simulink model "Thirtybussys_final"  (R2023b)
settings: Solver=VariableStepAuto  StartTime=0.0  StopTime=0.7  RelTol=1e-3
libraries: eePowerMeasurement x60, spsFourierLib x60, spsThreePhaseSeriesRLCBranchLib x41, spsThreePhaseVIMeasurementLib x30, spsThreePhaseSeriesRLCLoadLib x21, spsThreePhaseSourceLib x6, spsThreePhaseTransformerTwoWindingsLib x6, spsThreePhaseFaultLib x2, spspowerguiLib x1
(part 2 of 3)

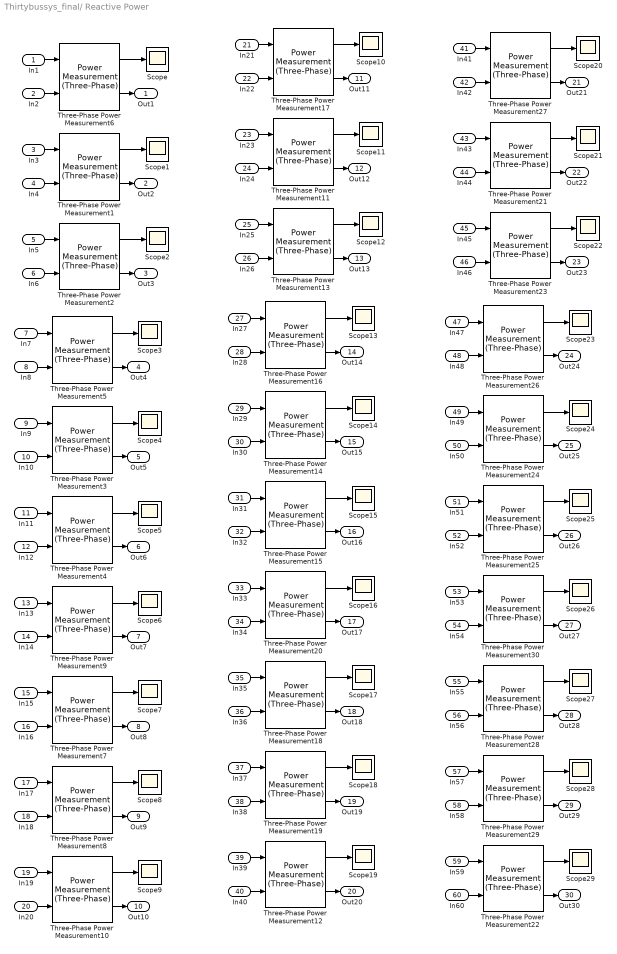
== system Thirtybussys_final/ Reactive Power ==
  In1 : Inport
  In2 : Inport  Port=2
  In3 : Inport  Port=3
  In4 : Inport  Port=4
  In5 : Inport  Port=5
  In6 : Inport  Port=6
  In7 : Inport  Port=7
  In8 : Inport  Port=8
  In9 : Inport  Port=9
  In10 : Inport  Port=10
  In11 : Inport  Port=11
  In12 : Inport  Port=12
  In13 : Inport  Port=13
  In14 : Inport  Port=14
  In15 : Inport  Port=15
  In16 : Inport  Port=16
  In17 : Inport  Port=17
  In18 : Inport  Port=18
  In19 : Inport  Port=19
  In20 : Inport  Port=20
  In21 : Inport  Port=21
  In22 : Inport  Port=22
  In23 : Inport  Port=23
  In24 : Inport  Port=24
  In25 : Inport  Port=25
  In26 : Inport  Port=26
  In27 : Inport  Port=27
  In28 : Inport  Port=28
  In29 : Inport  Port=29
  In30 : Inport  Port=30
  In31 : Inport  Port=31
  In32 : Inport  Port=32
  In33 : Inport  Port=33
  In34 : Inport  Port=34
  In35 : Inport  Port=35
  In36 : Inport  Port=36
  In37 : Inport  Port=37
  In38 : Inport  Port=38
  In39 : Inport  Port=39
  In40 : Inport  Port=40
  In41 : Inport  Port=41
  In42 : Inport  Port=42
  In43 : Inport  Port=43
  In44 : Inport  Port=44
  In45 : Inport  Port=45
  In46 : Inport  Port=46
  In47 : Inport  Port=47
  In48 : Inport  Port=48
  In49 : Inport  Port=49
  In50 : Inport  Port=50
  In51 : Inport  Port=51
  In52 : Inport  Port=52
  In53 : Inport  Port=53
  In54 : Inport  Port=54
  In55 : Inport  Port=55
  In56 : Inport  Port=56
  In57 : Inport  Port=57
  In58 : Inport  Port=58
  In59 : Inport  Port=59
  In60 : Inport  Port=60
  Scope{,1..29} (30 alike) : Scope
  Three-Phase Power Measurement{1..30} (30 alike) : eePowerMeasurement/Power Measurement (Three-Phase)  LabelModeActiveChoice=Continuous  F=60  K=0  Seq=Positive  Ts=0
  Out1 : Outport  VectorParamsAs1DForOutWhenUnconnected=off
  Out2 : Outport  Port=2  VectorParamsAs1DForOutWhenUnconnected=off
  Out3 : Outport  Port=3  VectorParamsAs1DForOutWhenUnconnected=off
  Out4 : Outport  Port=4  VectorParamsAs1DForOutWhenUnconnected=off
  Out5 : Outport  Port=5  VectorParamsAs1DForOutWhenUnconnected=off
  Out6 : Outport  Port=6  VectorParamsAs1DForOutWhenUnconnected=off
  Out7 : Outport  Port=7  VectorParamsAs1DForOutWhenUnconnected=off
  Out8 : Outport  Port=8  VectorParamsAs1DForOutWhenUnconnected=off
  Out9 : Outport  Port=9  VectorParamsAs1DForOutWhenUnconnected=off
  Out10 : Outport  Port=10  VectorParamsAs1DForOutWhenUnconnected=off
  Out11 : Outport  Port=11  VectorParamsAs1DForOutWhenUnconnected=off
  Out12 : Outport  Port=12  VectorParamsAs1DForOutWhenUnconnected=off
  Out13 : Outport  Port=13  VectorParamsAs1DForOutWhenUnconnected=off
  Out14 : Outport  Port=14  VectorParamsAs1DForOutWhenUnconnected=off
  Out15 : Outport  Port=15  VectorParamsAs1DForOutWhenUnconnected=off
  Out16 : Outport  Port=16  VectorParamsAs1DForOutWhenUnconnected=off
  Out17 : Outport  Port=17  VectorParamsAs1DForOutWhenUnconnected=off
  Out18 : Outport  Port=18  VectorParamsAs1DForOutWhenUnconnected=off
  Out19 : Outport  Port=19  VectorParamsAs1DForOutWhenUnconnected=off
  Out20 : Outport  Port=20  VectorParamsAs1DForOutWhenUnconnected=off
  Out21 : Outport  Port=21  VectorParamsAs1DForOutWhenUnconnected=off
  Out22 : Outport  Port=22  VectorParamsAs1DForOutWhenUnconnected=off
  Out23 : Outport  Port=23  VectorParamsAs1DForOutWhenUnconnected=off
  Out24 : Outport  Port=24  VectorParamsAs1DForOutWhenUnconnected=off
  Out25 : Outport  Port=25  VectorParamsAs1DForOutWhenUnconnected=off
  Out26 : Outport  Port=26  VectorParamsAs1DForOutWhenUnconnected=off
  Out27 : Outport  Port=27  VectorParamsAs1DForOutWhenUnconnected=off
  Out28 : Outport  Port=28  VectorParamsAs1DForOutWhenUnconnected=off
  Out29 : Outport  Port=29  VectorParamsAs1DForOutWhenUnconnected=off
  Out30 : Outport  Port=30  VectorParamsAs1DForOutWhenUnconnected=off
  wires:
  In2/1 -> Three-Phase Power Measurement6/2
  In1/1 -> Three-Phase Power Measurement6/1
  Three-Phase Power Measurement6/2 -> Out1/1
  Three-Phase Power Measurement6/1 -> Scope/1
  Three-Phase Power Measurement1/1 -> Scope1/1
  Three-Phase Power Measurement1/2 -> Out2/1
  In3/1 -> Three-Phase Power Measurement1/1
  In4/1 -> Three-Phase Power Measurement1/2
  In6/1 -> Three-Phase Power Measurement2/2
  In5/1 -> Three-Phase Power Measurement2/1
  Three-Phase Power Measurement2/2 -> Out3/1
  Three-Phase Power Measurement2/1 -> Scope2/1
  Three-Phase Power Measurement4/1 -> Scope5/1
  Three-Phase Power Measurement4/2 -> Out6/1
  In11/1 -> Three-Phase Power Measurement4/1
  In12/1 -> Three-Phase Power Measurement4/2
  In10/1 -> Three-Phase Power Measurement3/2
  In9/1 -> Three-Phase Power Measurement3/1
  Three-Phase Power Measurement3/2 -> Out5/1
  Three-Phase Power Measurement3/1 -> Scope4/1
  Three-Phase Power Measurement5/1 -> Scope3/1
  Three-Phase Power Measurement5/2 -> Out4/1
  In7/1 -> Three-Phase Power Measurement5/1
  In8/1 -> Three-Phase Power Measurement5/2
  In14/1 -> Three-Phase Power Measurement9/2
  In13/1 -> Three-Phase Power Measurement9/1
  Three-Phase Power Measurement9/2 -> Out7/1
  Three-Phase Power Measurement9/1 -> Scope6/1
  Three-Phase Power Measurement7/1 -> Scope7/1
  Three-Phase Power Measurement7/2 -> Out8/1
  In15/1 -> Three-Phase Power Measurement7/1
  In16/1 -> Three-Phase Power Measurement7/2
  In18/1 -> Three-Phase Power Measurement8/2
  In17/1 -> Three-Phase Power Measurement8/1
  Three-Phase Power Measurement8/2 -> Out9/1
  Three-Phase Power Measurement8/1 -> Scope8/1
  Three-Phase Power Measurement10/1 -> Scope9/1
  Three-Phase Power Measurement10/2 -> Out10/1
  In19/1 -> Three-Phase Power Measurement10/1
  In20/1 -> Three-Phase Power Measurement10/2
  In40/1 -> Three-Phase Power Measurement12/2
  In39/1 -> Three-Phase Power Measurement12/1
  Three-Phase Power Measurement12/2 -> Out20/1
  Three-Phase Power Measurement12/1 -> Scope19/1
  Three-Phase Power Measurement19/1 -> Scope18/1
  Three-Phase Power Measurement19/2 -> Out19/1
  In37/1 -> Three-Phase Power Measurement19/1
  In38/1 -> Three-Phase Power Measurement19/2
  In36/1 -> Three-Phase Power Measurement18/2
  In35/1 -> Three-Phase Power Measurement18/1
  Three-Phase Power Measurement18/2 -> Out18/1
  Three-Phase Power Measurement18/1 -> Scope17/1
  Three-Phase Power Measurement20/1 -> Scope16/1
  Three-Phase Power Measurement20/2 -> Out17/1
  In33/1 -> Three-Phase Power Measurement20/1
  In34/1 -> Three-Phase Power Measurement20/2
  In28/1 -> Three-Phase Power Measurement16/2
  In27/1 -> Three-Phase Power Measurement16/1
  Three-Phase Power Measurement16/2 -> Out14/1
  Three-Phase Power Measurement16/1 -> Scope13/1
  Three-Phase Power Measurement14/1 -> Scope14/1
  Three-Phase Power Measurement14/2 -> Out15/1
  In29/1 -> Three-Phase Power Measurement14/1
  In30/1 -> Three-Phase Power Measurement14/2
  In32/1 -> Three-Phase Power Measurement15/2
  In31/1 -> Three-Phase Power Measurement15/1
  Three-Phase Power Measurement15/2 -> Out16/1
  Three-Phase Power Measurement15/1 -> Scope15/1
  Three-Phase Power Measurement13/1 -> Scope12/1
  Three-Phase Power Measurement13/2 -> Out13/1
  In25/1 -> Three-Phase Power Measurement13/1
  In26/1 -> Three-Phase Power Measurement13/2
  In24/1 -> Three-Phase Power Measurement11/2
  In23/1 -> Three-Phase Power Measurement11/1
  Three-Phase Power Measurement11/2 -> Out12/1
  Three-Phase Power Measurement11/1 -> Scope11/1
  Three-Phase Power Measurement17/1 -> Scope10/1
  Three-Phase Power Measurement17/2 -> Out11/1
  In21/1 -> Three-Phase Power Measurement17/1
  In22/1 -> Three-Phase Power Measurement17/2
  In42/1 -> Three-Phase Power Measurement27/2
  In41/1 -> Three-Phase Power Measurement27/1
  Three-Phase Power Measurement27/2 -> Out21/1
  Three-Phase Power Measurement27/1 -> Scope20/1
  Three-Phase Power Measurement21/1 -> Scope21/1
  Three-Phase Power Measurement21/2 -> Out22/1
  In43/1 -> Three-Phase Power Measurement21/1
  In44/1 -> Three-Phase Power Measurement21/2
  In46/1 -> Three-Phase Power Measurement23/2
  In45/1 -> Three-Phase Power Measurement23/1
  Three-Phase Power Measurement23/2 -> Out23/1
  Three-Phase Power Measurement23/1 -> Scope22/1
  Three-Phase Power Measurement25/1 -> Scope25/1
  Three-Phase Power Measurement25/2 -> Out26/1
  In51/1 -> Three-Phase Power Measurement25/1
  In52/1 -> Three-Phase Power Measurement25/2
  In50/1 -> Three-Phase Power Measurement24/2
  In49/1 -> Three-Phase Power Measurement24/1
  Three-Phase Power Measurement24/2 -> Out25/1
  Three-Phase Power Measurement24/1 -> Scope24/1
  Three-Phase Power Measurement26/1 -> Scope23/1
  Three-Phase Power Measurement26/2 -> Out24/1
  In47/1 -> Three-Phase Power Measurement26/1
  In48/1 -> Three-Phase Power Measurement26/2
  In54/1 -> Three-Phase Power Measurement30/2
  In53/1 -> Three-Phase Power Measurement30/1
  Three-Phase Power Measurement30/2 -> Out27/1
  Three-Phase Power Measurement30/1 -> Scope26/1
  Three-Phase Power Measurement28/1 -> Scope27/1
  Three-Phase Power Measurement28/2 -> Out28/1
  In55/1 -> Three-Phase Power Measurement28/1
  In56/1 -> Three-Phase Power Measurement28/2
  In58/1 -> Three-Phase Power Measurement29/2
  In57/1 -> Three-Phase Power Measurement29/1
  Three-Phase Power Measurement29/2 -> Out29/1
  Three-Phase Power Measurement29/1 -> Scope28/1
  Three-Phase Power Measurement22/1 -> Scope29/1
  Three-Phase Power Measurement22/2 -> Out30/1
  In59/1 -> Three-Phase Power Measurement22/1
  In60/1 -> Three-Phase Power Measurement22/2

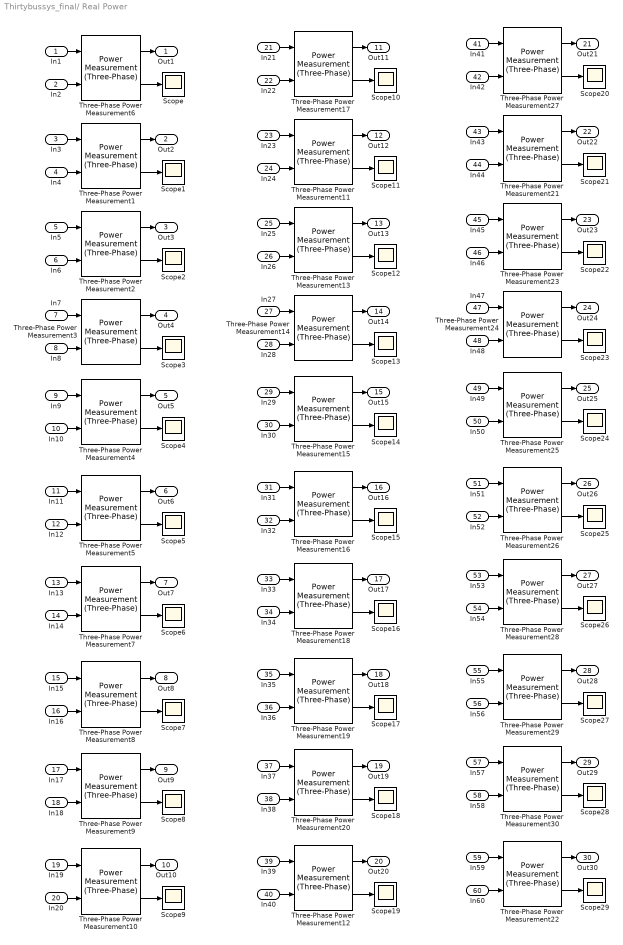
== system Thirtybussys_final/ Real Power ==
  In1 : Inport
  In2 : Inport  Port=2
  In3 : Inport  Port=3
  In4 : Inport  Port=4
  In5 : Inport  Port=5
  In6 : Inport  Port=6
  In7 : Inport  Port=7
  In8 : Inport  Port=8
  In9 : Inport  Port=9
  In10 : Inport  Port=10
  In11 : Inport  Port=11
  In12 : Inport  Port=12
  In13 : Inport  Port=13
  In14 : Inport  Port=14
  In15 : Inport  Port=15
  In16 : Inport  Port=16
  In17 : Inport  Port=17
  In18 : Inport  Port=18
  In19 : Inport  Port=19
  In20 : Inport  Port=20
  In21 : Inport  Port=21
  In22 : Inport  Port=22
  In23 : Inport  Port=23
  In24 : Inport  Port=24
  In25 : Inport  Port=25
  In26 : Inport  Port=26
  In27 : Inport  Port=27
  In28 : Inport  Port=28
  In29 : Inport  Port=29
  In30 : Inport  Port=30
  In31 : Inport  Port=31
  In32 : Inport  Port=32
  In33 : Inport  Port=33
  In34 : Inport  Port=34
  In35 : Inport  Port=35
  In36 : Inport  Port=36
  In37 : Inport  Port=37
  In38 : Inport  Port=38
  In39 : Inport  Port=39
  In40 : Inport  Port=40
  In41 : Inport  Port=41
  In42 : Inport  Port=42
  In43 : Inport  Port=43
  In44 : Inport  Port=44
  In45 : Inport  Port=45
  In46 : Inport  Port=46
  In47 : Inport  Port=47
  In48 : Inport  Port=48
  In49 : Inport  Port=49
  In50 : Inport  Port=50
  In51 : Inport  Port=51
  In52 : Inport  Port=52
  In53 : Inport  Port=53
  In54 : Inport  Port=54
  In55 : Inport  Port=55
  In56 : Inport  Port=56
  In57 : Inport  Port=57
  In58 : Inport  Port=58
  In59 : Inport  Port=59
  In60 : Inport  Port=60
  Scope{,1..29} (30 alike) : Scope
  Three-Phase Power Measurement{1..30} (30 alike) : eePowerMeasurement/Power Measurement (Three-Phase)  LabelModeActiveChoice=Continuous  F=60  K=0  Seq=Positive  Ts=0
  Out1 : Outport  VectorParamsAs1DForOutWhenUnconnected=off
  Out2 : Outport  Port=2  VectorParamsAs1DForOutWhenUnconnected=off
  Out3 : Outport  Port=3  VectorParamsAs1DForOutWhenUnconnected=off
  Out4 : Outport  Port=4  VectorParamsAs1DForOutWhenUnconnected=off
  Out5 : Outport  Port=5  VectorParamsAs1DForOutWhenUnconnected=off
  Out6 : Outport  Port=6  VectorParamsAs1DForOutWhenUnconnected=off
  Out7 : Outport  Port=7  VectorParamsAs1DForOutWhenUnconnected=off
  Out8 : Outport  Port=8  VectorParamsAs1DForOutWhenUnconnected=off
  Out9 : Outport  Port=9  VectorParamsAs1DForOutWhenUnconnected=off
  Out10 : Outport  Port=10  VectorParamsAs1DForOutWhenUnconnected=off
  Out11 : Outport  Port=11  VectorParamsAs1DForOutWhenUnconnected=off
  Out12 : Outport  Port=12  VectorParamsAs1DForOutWhenUnconnected=off
  Out13 : Outport  Port=13  VectorParamsAs1DForOutWhenUnconnected=off
  Out14 : Outport  Port=14  VectorParamsAs1DForOutWhenUnconnected=off
  Out15 : Outport  Port=15  VectorParamsAs1DForOutWhenUnconnected=off
  Out16 : Outport  Port=16  VectorParamsAs1DForOutWhenUnconnected=off
  Out17 : Outport  Port=17  VectorParamsAs1DForOutWhenUnconnected=off
  Out18 : Outport  Port=18  VectorParamsAs1DForOutWhenUnconnected=off
  Out19 : Outport  Port=19  VectorParamsAs1DForOutWhenUnconnected=off
  Out20 : Outport  Port=20  VectorParamsAs1DForOutWhenUnconnected=off
  Out21 : Outport  Port=21  VectorParamsAs1DForOutWhenUnconnected=off
  Out22 : Outport  Port=22  VectorParamsAs1DForOutWhenUnconnected=off
  Out23 : Outport  Port=23  VectorParamsAs1DForOutWhenUnconnected=off
  Out24 : Outport  Port=24  VectorParamsAs1DForOutWhenUnconnected=off
  Out25 : Outport  Port=25  VectorParamsAs1DForOutWhenUnconnected=off
  Out26 : Outport  Port=26  VectorParamsAs1DForOutWhenUnconnected=off
  Out27 : Outport  Port=27  VectorParamsAs1DForOutWhenUnconnected=off
  Out28 : Outport  Port=28  VectorParamsAs1DForOutWhenUnconnected=off
  Out29 : Outport  Port=29  VectorParamsAs1DForOutWhenUnconnected=off
  Out30 : Outport  Port=30  VectorParamsAs1DForOutWhenUnconnected=off
  wires:
  In1/1 -> Three-Phase Power Measurement6/1
  In2/1 -> Three-Phase Power Measurement6/2
  Three-Phase Power Measurement6/1 -> Out1/1
  Three-Phase Power Measurement6/2 -> Scope/1
  Three-Phase Power Measurement1/2 -> Scope1/1
  Three-Phase Power Measurement1/1 -> Out2/1
  In4/1 -> Three-Phase Power Measurement1/2
  In3/1 -> Three-Phase Power Measurement1/1
  In5/1 -> Three-Phase Power Measurement2/1
  In6/1 -> Three-Phase Power Measurement2/2
  Three-Phase Power Measurement2/1 -> Out3/1
  Three-Phase Power Measurement2/2 -> Scope2/1
  Three-Phase Power Measurement3/2 -> Scope3/1
  Three-Phase Power Measurement3/1 -> Out4/1
  In8/1 -> Three-Phase Power Measurement3/2
  In7/1 -> Three-Phase Power Measurement3/1
  In9/1 -> Three-Phase Power Measurement4/1
  In10/1 -> Three-Phase Power Measurement4/2
  Three-Phase Power Measurement4/1 -> Out5/1
  Three-Phase Power Measurement4/2 -> Scope4/1
  Three-Phase Power Measurement5/2 -> Scope5/1
  Three-Phase Power Measurement5/1 -> Out6/1
  In12/1 -> Three-Phase Power Measurement5/2
  In11/1 -> Three-Phase Power Measurement5/1
  In13/1 -> Three-Phase Power Measurement7/1
  In14/1 -> Three-Phase Power Measurement7/2
  Three-Phase Power Measurement7/1 -> Out7/1
  Three-Phase Power Measurement7/2 -> Scope6/1
  Three-Phase Power Measurement8/2 -> Scope7/1
  Three-Phase Power Measurement8/1 -> Out8/1
  In16/1 -> Three-Phase Power Measurement8/2
  In15/1 -> Three-Phase Power Measurement8/1
  In19/1 -> Three-Phase Power Measurement10/1
  In20/1 -> Three-Phase Power Measurement10/2
  Three-Phase Power Measurement10/1 -> Out10/1
  Three-Phase Power Measurement10/2 -> Scope9/1
  Three-Phase Power Measurement9/2 -> Scope8/1
  Three-Phase Power Measurement9/1 -> Out9/1
  In18/1 -> Three-Phase Power Measurement9/2
  In17/1 -> Three-Phase Power Measurement9/1
  In37/1 -> Three-Phase Power Measurement20/1
  In38/1 -> Three-Phase Power Measurement20/2
  Three-Phase Power Measurement20/1 -> Out19/1
  Three-Phase Power Measurement20/2 -> Scope18/1
  Three-Phase Power Measurement12/2 -> Scope19/1
  Three-Phase Power Measurement12/1 -> Out20/1
  In40/1 -> Three-Phase Power Measurement12/2
  In39/1 -> Three-Phase Power Measurement12/1
  In35/1 -> Three-Phase Power Measurement19/1
  In36/1 -> Three-Phase Power Measurement19/2
  Three-Phase Power Measurement19/1 -> Out18/1
  Three-Phase Power Measurement19/2 -> Scope17/1
  Three-Phase Power Measurement18/2 -> Scope16/1
  Three-Phase Power Measurement18/1 -> Out17/1
  In34/1 -> Three-Phase Power Measurement18/2
  In33/1 -> Three-Phase Power Measurement18/1
  In31/1 -> Three-Phase Power Measurement16/1
  In32/1 -> Three-Phase Power Measurement16/2
  Three-Phase Power Measurement16/1 -> Out16/1
  Three-Phase Power Measurement16/2 -> Scope15/1
  Three-Phase Power Measurement15/2 -> Scope14/1
  Three-Phase Power Measurement15/1 -> Out15/1
  In30/1 -> Three-Phase Power Measurement15/2
  In29/1 -> Three-Phase Power Measurement15/1
  In27/1 -> Three-Phase Power Measurement14/1
  In28/1 -> Three-Phase Power Measurement14/2
  Three-Phase Power Measurement14/1 -> Out14/1
  Three-Phase Power Measurement14/2 -> Scope13/1
  Three-Phase Power Measurement13/2 -> Scope12/1
  Three-Phase Power Measurement13/1 -> Out13/1
  In26/1 -> Three-Phase Power Measurement13/2
  In25/1 -> Three-Phase Power Measurement13/1
  In23/1 -> Three-Phase Power Measurement11/1
  In24/1 -> Three-Phase Power Measurement11/2
  Three-Phase Power Measurement11/1 -> Out12/1
  Three-Phase Power Measurement11/2 -> Scope11/1
  Three-Phase Power Measurement17/2 -> Scope10/1
  Three-Phase Power Measurement17/1 -> Out11/1
  In22/1 -> Three-Phase Power Measurement17/2
  In21/1 -> Three-Phase Power Measurement17/1
  In41/1 -> Three-Phase Power Measurement27/1
  In42/1 -> Three-Phase Power Measurement27/2
  Three-Phase Power Measurement27/1 -> Out21/1
  Three-Phase Power Measurement27/2 -> Scope20/1
  Three-Phase Power Measurement21/2 -> Scope21/1
  Three-Phase Power Measurement21/1 -> Out22/1
  In44/1 -> Three-Phase Power Measurement21/2
  In43/1 -> Three-Phase Power Measurement21/1
  In45/1 -> Three-Phase Power Measurement23/1
  In46/1 -> Three-Phase Power Measurement23/2
  Three-Phase Power Measurement23/1 -> Out23/1
  Three-Phase Power Measurement23/2 -> Scope22/1
  Three-Phase Power Measurement24/2 -> Scope23/1
  Three-Phase Power Measurement24/1 -> Out24/1
  In48/1 -> Three-Phase Power Measurement24/2
  In47/1 -> Three-Phase Power Measurement24/1
  In49/1 -> Three-Phase Power Measurement25/1
  In50/1 -> Three-Phase Power Measurement25/2
  Three-Phase Power Measurement25/1 -> Out25/1
  Three-Phase Power Measurement25/2 -> Scope24/1
  Three-Phase Power Measurement26/2 -> Scope25/1
  Three-Phase Power Measurement26/1 -> Out26/1
  In52/1 -> Three-Phase Power Measurement26/2
  In51/1 -> Three-Phase Power Measurement26/1
  In53/1 -> Three-Phase Power Measurement28/1
  In54/1 -> Three-Phase Power Measurement28/2
  Three-Phase Power Measurement28/1 -> Out27/1
  Three-Phase Power Measurement28/2 -> Scope26/1
  Three-Phase Power Measurement29/2 -> Scope27/1
  Three-Phase Power Measurement29/1 -> Out28/1
  In56/1 -> Three-Phase Power Measurement29/2
  In55/1 -> Three-Phase Power Measurement29/1
  In59/1 -> Three-Phase Power Measurement22/1
  In60/1 -> Three-Phase Power Measurement22/2
  Three-Phase Power Measurement22/1 -> Out30/1
  Three-Phase Power Measurement22/2 -> Scope29/1
  Three-Phase Power Measurement30/2 -> Scope28/1
  Three-Phase Power Measurement30/1 -> Out29/1
  In58/1 -> Three-Phase Power Measurement30/2
  In57/1 -> Three-Phase Power Measurement30/1

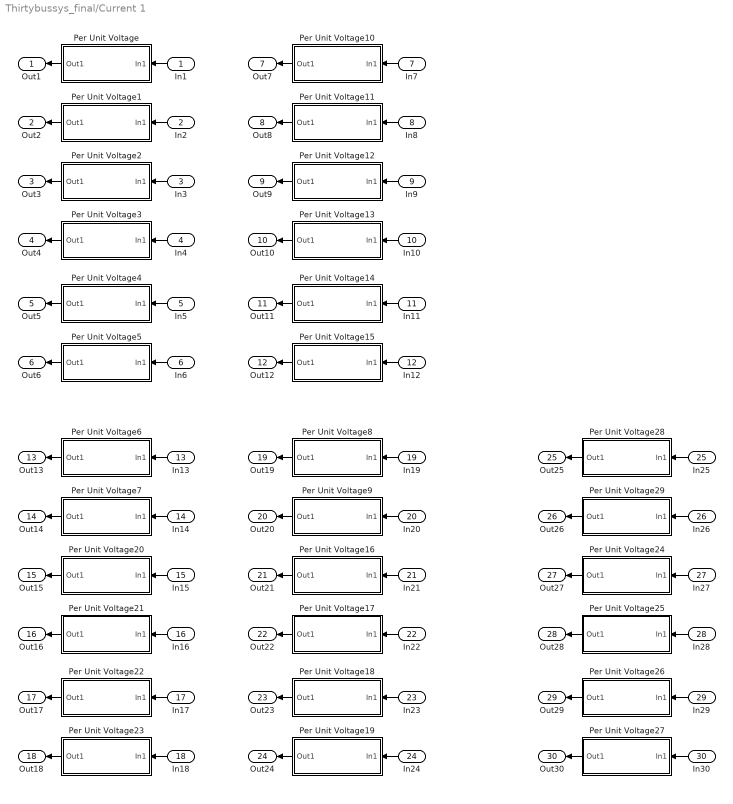
== system Thirtybussys_final/Current 1 ==
  In1 : Inport
  In2 : Inport  Port=2
  In3 : Inport  Port=3
  In4 : Inport  Port=4
  In5 : Inport  Port=5
  In6 : Inport  Port=6
  In7 : Inport  Port=7
  In8 : Inport  Port=8
  In9 : Inport  Port=9
  In10 : Inport  Port=10
  In11 : Inport  Port=11
  In12 : Inport  Port=12
  In13 : Inport  Port=13
  In14 : Inport  Port=14
  In15 : Inport  Port=15
  In16 : Inport  Port=16
  In17 : Inport  Port=17
  In18 : Inport  Port=18
  In19 : Inport  Port=19
  In20 : Inport  Port=20
  In21 : Inport  Port=21
  In22 : Inport  Port=22
  In23 : Inport  Port=23
  In24 : Inport  Port=24
  In25 : Inport  Port=25
  In26 : Inport  Port=26
  In27 : Inport  Port=27
  In28 : Inport  Port=28
  In29 : Inport  Port=29
  In30 : Inport  Port=30
  Per Unit Voltage : Subsystem
  Per Unit Voltage1 : Subsystem
  Per Unit Voltage10 : Subsystem
  Per Unit Voltage11 : Subsystem
  Per Unit Voltage12 : Subsystem
  Per Unit Voltage13 : Subsystem
  Per Unit Voltage14 : Subsystem
  Per Unit Voltage15 : Subsystem
  Per Unit Voltage16 : Subsystem
  Per Unit Voltage17 : Subsystem
  Per Unit Voltage18 : Subsystem
  Per Unit Voltage19 : Subsystem
  Per Unit Voltage2 : Subsystem
  Per Unit Voltage20 : Subsystem
  Per Unit Voltage21 : Subsystem
  Per Unit Voltage22 : Subsystem
  Per Unit Voltage23 : Subsystem
  Per Unit Voltage24 : Subsystem
  Per Unit Voltage25 : Subsystem
  Per Unit Voltage26 : Subsystem
  Per Unit Voltage27 : Subsystem
  Per Unit Voltage28 : Subsystem
  Per Unit Voltage29 : Subsystem
  Per Unit Voltage3 : Subsystem
  Per Unit Voltage4 : Subsystem
  Per Unit Voltage5 : Subsystem
  Per Unit Voltage6 : Subsystem
  Per Unit Voltage7 : Subsystem
  Per Unit Voltage8 : Subsystem
  Per Unit Voltage9 : Subsystem
  Out1 : Outport  VectorParamsAs1DForOutWhenUnconnected=off
  Out2 : Outport  Port=2  VectorParamsAs1DForOutWhenUnconnected=off
  Out3 : Outport  Port=3  VectorParamsAs1DForOutWhenUnconnected=off
  Out4 : Outport  Port=4  VectorParamsAs1DForOutWhenUnconnected=off
  Out5 : Outport  Port=5  VectorParamsAs1DForOutWhenUnconnected=off
  Out6 : Outport  Port=6  VectorParamsAs1DForOutWhenUnconnected=off
  Out7 : Outport  Port=7  VectorParamsAs1DForOutWhenUnconnected=off
  Out8 : Outport  Port=8  VectorParamsAs1DForOutWhenUnconnected=off
  Out9 : Outport  Port=9  VectorParamsAs1DForOutWhenUnconnected=off
  Out10 : Outport  Port=10  VectorParamsAs1DForOutWhenUnconnected=off
  Out11 : Outport  Port=11  VectorParamsAs1DForOutWhenUnconnected=off
  Out12 : Outport  Port=12  VectorParamsAs1DForOutWhenUnconnected=off
  Out13 : Outport  Port=13  VectorParamsAs1DForOutWhenUnconnected=off
  Out14 : Outport  Port=14  VectorParamsAs1DForOutWhenUnconnected=off
  Out15 : Outport  Port=15  VectorParamsAs1DForOutWhenUnconnected=off
  Out16 : Outport  Port=16  VectorParamsAs1DForOutWhenUnconnected=off
  Out17 : Outport  Port=17  VectorParamsAs1DForOutWhenUnconnected=off
  Out18 : Outport  Port=18  VectorParamsAs1DForOutWhenUnconnected=off
  Out19 : Outport  Port=19  VectorParamsAs1DForOutWhenUnconnected=off
  Out20 : Outport  Port=20  VectorParamsAs1DForOutWhenUnconnected=off
  Out21 : Outport  Port=21  VectorParamsAs1DForOutWhenUnconnected=off
  Out22 : Outport  Port=22  VectorParamsAs1DForOutWhenUnconnected=off
  Out23 : Outport  Port=23  VectorParamsAs1DForOutWhenUnconnected=off
  Out24 : Outport  Port=24  VectorParamsAs1DForOutWhenUnconnected=off
  Out25 : Outport  Port=25  VectorParamsAs1DForOutWhenUnconnected=off
  Out26 : Outport  Port=26  VectorParamsAs1DForOutWhenUnconnected=off
  Out27 : Outport  Port=27  VectorParamsAs1DForOutWhenUnconnected=off
  Out28 : Outport  Port=28  VectorParamsAs1DForOutWhenUnconnected=off
  Out29 : Outport  Port=29  VectorParamsAs1DForOutWhenUnconnected=off
  Out30 : Outport  Port=30  VectorParamsAs1DForOutWhenUnconnected=off
  wires:
  Per Unit Voltage2/1(Out1) -> Out3/1
  In2/1 -> Per Unit Voltage1/1(In1)
  Per Unit Voltage5/1(Out1) -> Out6/1
  In5/1 -> Per Unit Voltage4/1(In1)
  Per Unit Voltage1/1(Out1) -> Out2/1
  In1/1 -> Per Unit Voltage/1(In1)
  Per Unit Voltage3/1(Out1) -> Out4/1
  Per Unit Voltage/1(Out1) -> Out1/1
  In4/1 -> Per Unit Voltage3/1(In1)
  In3/1 -> Per Unit Voltage2/1(In1)
  Per Unit Voltage4/1(Out1) -> Out5/1
  In6/1 -> Per Unit Voltage5/1(In1)
  In7/1 -> Per Unit Voltage10/1(In1)
  Per Unit Voltage15/1(Out1) -> Out12/1
  Per Unit Voltage14/1(Out1) -> Out11/1
  Per Unit Voltage11/1(Out1) -> Out8/1
  In12/1 -> Per Unit Voltage15/1(In1)
  Per Unit Voltage10/1(Out1) -> Out7/1
  Per Unit Voltage12/1(Out1) -> Out9/1
  In10/1 -> Per Unit Voltage13/1(In1)
  Per Unit Voltage13/1(Out1) -> Out10/1
  In9/1 -> Per Unit Voltage12/1(In1)
  In11/1 -> Per Unit Voltage14/1(In1)
  In8/1 -> Per Unit Voltage11/1(In1)
  In20/1 -> Per Unit Voltage9/1(In1)
  In23/1 -> Per Unit Voltage18/1(In1)
  In21/1 -> Per Unit Voltage16/1(In1)
  Per Unit Voltage17/1(Out1) -> Out22/1
  In22/1 -> Per Unit Voltage17/1(In1)
  Per Unit Voltage16/1(Out1) -> Out21/1
  Per Unit Voltage8/1(Out1) -> Out19/1
  In24/1 -> Per Unit Voltage19/1(In1)
  Per Unit Voltage9/1(Out1) -> Out20/1
  Per Unit Voltage18/1(Out1) -> Out23/1
  Per Unit Voltage19/1(Out1) -> Out24/1
  In19/1 -> Per Unit Voltage8/1(In1)
  In18/1 -> Per Unit Voltage23/1(In1)
  Per Unit Voltage22/1(Out1) -> Out17/1
  In15/1 -> Per Unit Voltage20/1(In1)
  In16/1 -> Per Unit Voltage21/1(In1)
  Per Unit Voltage6/1(Out1) -> Out13/1
  Per Unit Voltage21/1(Out1) -> Out16/1
  In13/1 -> Per Unit Voltage6/1(In1)
  Per Unit Voltage7/1(Out1) -> Out14/1
  In17/1 -> Per Unit Voltage22/1(In1)
  Per Unit Voltage23/1(Out1) -> Out18/1
  In14/1 -> Per Unit Voltage7/1(In1)
  Per Unit Voltage20/1(Out1) -> Out15/1
  Per Unit Voltage24/1(Out1) -> Out27/1
  In26/1 -> Per Unit Voltage29/1(In1)
  Per Unit Voltage27/1(Out1) -> Out30/1
  In29/1 -> Per Unit Voltage26/1(In1)
  Per Unit Voltage29/1(Out1) -> Out26/1
  In25/1 -> Per Unit Voltage28/1(In1)
  Per Unit Voltage25/1(Out1) -> Out28/1
  Per Unit Voltage28/1(Out1) -> Out25/1
  In28/1 -> Per Unit Voltage25/1(In1)
  In27/1 -> Per Unit Voltage24/1(In1)
  Per Unit Voltage26/1(Out1) -> Out29/1
  In30/1 -> Per Unit Voltage27/1(In1)

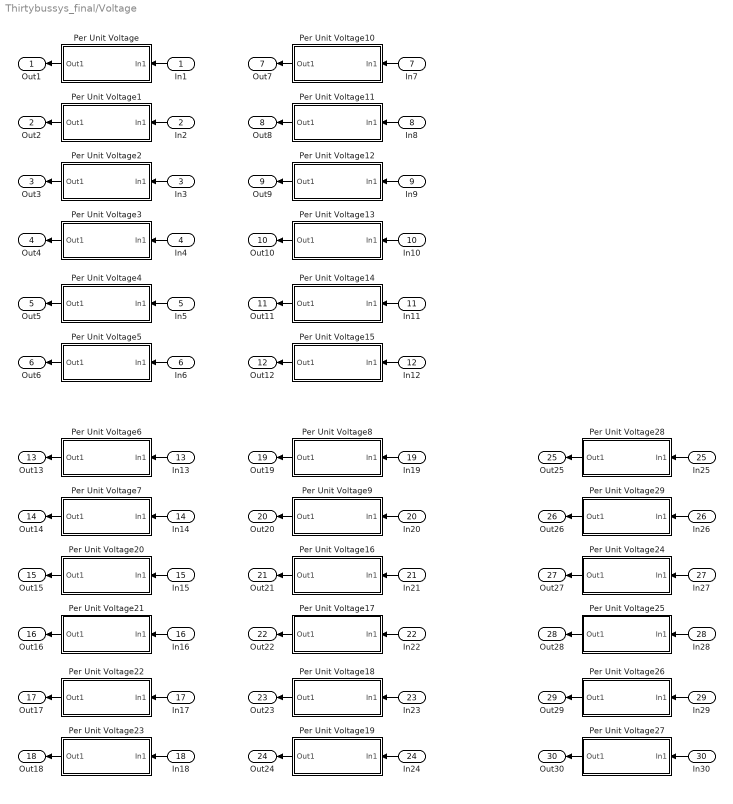
== system Thirtybussys_final/Voltage  ==
  In1 : Inport
  In2 : Inport  Port=2
  In3 : Inport  Port=3
  In4 : Inport  Port=4
  In5 : Inport  Port=5
  In6 : Inport  Port=6
  In7 : Inport  Port=7
  In8 : Inport  Port=8
  In9 : Inport  Port=9
  In10 : Inport  Port=10
  In11 : Inport  Port=11
  In12 : Inport  Port=12
  In13 : Inport  Port=13
  In14 : Inport  Port=14
  In15 : Inport  Port=15
  In16 : Inport  Port=16
  In17 : Inport  Port=17
  In18 : Inport  Port=18
  In19 : Inport  Port=19
  In20 : Inport  Port=20
  In21 : Inport  Port=21
  In22 : Inport  Port=22
  In23 : Inport  Port=23
  In24 : Inport  Port=24
  In25 : Inport  Port=25
  In26 : Inport  Port=26
  In27 : Inport  Port=27
  In28 : Inport  Port=28
  In29 : Inport  Port=29
  In30 : Inport  Port=30
  Per Unit Voltage : Subsystem
  Per Unit Voltage1 : Subsystem
  Per Unit Voltage10 : Subsystem
  Per Unit Voltage11 : Subsystem
  Per Unit Voltage12 : Subsystem
  Per Unit Voltage13 : Subsystem
  Per Unit Voltage14 : Subsystem
  Per Unit Voltage15 : Subsystem
  Per Unit Voltage16 : Subsystem
  Per Unit Voltage17 : Subsystem
  Per Unit Voltage18 : Subsystem
  Per Unit Voltage19 : Subsystem
  Per Unit Voltage2 : Subsystem
  Per Unit Voltage20 : Subsystem
  Per Unit Voltage21 : Subsystem
  Per Unit Voltage22 : Subsystem
  Per Unit Voltage23 : Subsystem
  Per Unit Voltage24 : Subsystem
  Per Unit Voltage25 : Subsystem
  Per Unit Voltage26 : Subsystem
  Per Unit Voltage27 : Subsystem
  Per Unit Voltage28 : Subsystem
  Per Unit Voltage29 : Subsystem
  Per Unit Voltage3 : Subsystem
  Per Unit Voltage4 : Subsystem
  Per Unit Voltage5 : Subsystem
  Per Unit Voltage6 : Subsystem
  Per Unit Voltage7 : Subsystem
  Per Unit Voltage8 : Subsystem
  Per Unit Voltage9 : Subsystem
  Out1 : Outport  VectorParamsAs1DForOutWhenUnconnected=off
  Out2 : Outport  Port=2  VectorParamsAs1DForOutWhenUnconnected=off
  Out3 : Outport  Port=3  VectorParamsAs1DForOutWhenUnconnected=off
  Out4 : Outport  Port=4  VectorParamsAs1DForOutWhenUnconnected=off
  Out5 : Outport  Port=5  VectorParamsAs1DForOutWhenUnconnected=off
  Out6 : Outport  Port=6  VectorParamsAs1DForOutWhenUnconnected=off
  Out7 : Outport  Port=7  VectorParamsAs1DForOutWhenUnconnected=off
  Out8 : Outport  Port=8  VectorParamsAs1DForOutWhenUnconnected=off
  Out9 : Outport  Port=9  VectorParamsAs1DForOutWhenUnconnected=off
  Out10 : Outport  Port=10  VectorParamsAs1DForOutWhenUnconnected=off
  Out11 : Outport  Port=11  VectorParamsAs1DForOutWhenUnconnected=off
  Out12 : Outport  Port=12  VectorParamsAs1DForOutWhenUnconnected=off
  Out13 : Outport  Port=13  VectorParamsAs1DForOutWhenUnconnected=off
  Out14 : Outport  Port=14  VectorParamsAs1DForOutWhenUnconnected=off
  Out15 : Outport  Port=15  VectorParamsAs1DForOutWhenUnconnected=off
  Out16 : Outport  Port=16  VectorParamsAs1DForOutWhenUnconnected=off
  Out17 : Outport  Port=17  VectorParamsAs1DForOutWhenUnconnected=off
  Out18 : Outport  Port=18  VectorParamsAs1DForOutWhenUnconnected=off
  Out19 : Outport  Port=19  VectorParamsAs1DForOutWhenUnconnected=off
  Out20 : Outport  Port=20  VectorParamsAs1DForOutWhenUnconnected=off
  Out21 : Outport  Port=21  VectorParamsAs1DForOutWhenUnconnected=off
  Out22 : Outport  Port=22  VectorParamsAs1DForOutWhenUnconnected=off
  Out23 : Outport  Port=23  VectorParamsAs1DForOutWhenUnconnected=off
  Out24 : Outport  Port=24  VectorParamsAs1DForOutWhenUnconnected=off
  Out25 : Outport  Port=25  VectorParamsAs1DForOutWhenUnconnected=off
  Out26 : Outport  Port=26  VectorParamsAs1DForOutWhenUnconnected=off
  Out27 : Outport  Port=27  VectorParamsAs1DForOutWhenUnconnected=off
  Out28 : Outport  Port=28  VectorParamsAs1DForOutWhenUnconnected=off
  Out29 : Outport  Port=29  VectorParamsAs1DForOutWhenUnconnected=off
  Out30 : Outport  Port=30  VectorParamsAs1DForOutWhenUnconnected=off
  wires:
  Per Unit Voltage2/1(Out1) -> Out3/1
  In2/1 -> Per Unit Voltage1/1(In1)
  Per Unit Voltage5/1(Out1) -> Out6/1
  In5/1 -> Per Unit Voltage4/1(In1)
  Per Unit Voltage1/1(Out1) -> Out2/1
  In1/1 -> Per Unit Voltage/1(In1)
  Per Unit Voltage3/1(Out1) -> Out4/1
  Per Unit Voltage/1(Out1) -> Out1/1
  In4/1 -> Per Unit Voltage3/1(In1)
  In3/1 -> Per Unit Voltage2/1(In1)
  Per Unit Voltage4/1(Out1) -> Out5/1
  In6/1 -> Per Unit Voltage5/1(In1)
  In7/1 -> Per Unit Voltage10/1(In1)
  Per Unit Voltage15/1(Out1) -> Out12/1
  Per Unit Voltage14/1(Out1) -> Out11/1
  Per Unit Voltage11/1(Out1) -> Out8/1
  In12/1 -> Per Unit Voltage15/1(In1)
  Per Unit Voltage10/1(Out1) -> Out7/1
  Per Unit Voltage12/1(Out1) -> Out9/1
  In10/1 -> Per Unit Voltage13/1(In1)
  Per Unit Voltage13/1(Out1) -> Out10/1
  In9/1 -> Per Unit Voltage12/1(In1)
  In11/1 -> Per Unit Voltage14/1(In1)
  In8/1 -> Per Unit Voltage11/1(In1)
  In20/1 -> Per Unit Voltage9/1(In1)
  In23/1 -> Per Unit Voltage18/1(In1)
  In21/1 -> Per Unit Voltage16/1(In1)
  Per Unit Voltage17/1(Out1) -> Out22/1
  In22/1 -> Per Unit Voltage17/1(In1)
  Per Unit Voltage16/1(Out1) -> Out21/1
  Per Unit Voltage8/1(Out1) -> Out19/1
  In24/1 -> Per Unit Voltage19/1(In1)
  Per Unit Voltage9/1(Out1) -> Out20/1
  Per Unit Voltage18/1(Out1) -> Out23/1
  Per Unit Voltage19/1(Out1) -> Out24/1
  In19/1 -> Per Unit Voltage8/1(In1)
  In18/1 -> Per Unit Voltage23/1(In1)
  Per Unit Voltage22/1(Out1) -> Out17/1
  In15/1 -> Per Unit Voltage20/1(In1)
  In16/1 -> Per Unit Voltage21/1(In1)
  Per Unit Voltage6/1(Out1) -> Out13/1
  Per Unit Voltage21/1(Out1) -> Out16/1
  In13/1 -> Per Unit Voltage6/1(In1)
  Per Unit Voltage7/1(Out1) -> Out14/1
  In17/1 -> Per Unit Voltage22/1(In1)
  Per Unit Voltage23/1(Out1) -> Out18/1
  In14/1 -> Per Unit Voltage7/1(In1)
  Per Unit Voltage20/1(Out1) -> Out15/1
  Per Unit Voltage24/1(Out1) -> Out27/1
  In26/1 -> Per Unit Voltage29/1(In1)
  Per Unit Voltage27/1(Out1) -> Out30/1
  In29/1 -> Per Unit Voltage26/1(In1)
  Per Unit Voltage29/1(Out1) -> Out26/1
  In25/1 -> Per Unit Voltage28/1(In1)
  Per Unit Voltage25/1(Out1) -> Out28/1
  Per Unit Voltage28/1(Out1) -> Out25/1
  In28/1 -> Per Unit Voltage25/1(In1)
  In27/1 -> Per Unit Voltage24/1(In1)
  Per Unit Voltage26/1(Out1) -> Out29/1
  In30/1 -> Per Unit Voltage27/1(In1)

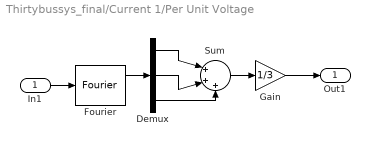
== system Thirtybussys_final/Current 1/Per Unit Voltage ==
  In1 : Inport
  Demux : Demux  Outputs=3
  Fourier : spsFourierLib/Fourier  Freq=60  n=1  InInit=[0, 0]  Ts=50e-6
  Gain : Gain  Gain=1/3
  Sum : Sum  Inputs=|+++
  Out1 : Outport  VectorParamsAs1DForOutWhenUnconnected=off
  wires:
  In1/1 -> Fourier/1
  Gain/1 -> Out1/1
  Fourier/1 -> Demux/1
  Demux/1 -> Sum/1
  Demux/2 -> Sum/2
  Demux/3 -> Sum/3
  Sum/1 -> Gain/1

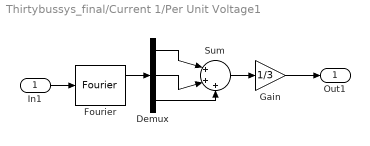
== system Thirtybussys_final/Current 1/Per Unit Voltage1 ==
  In1 : Inport
  Demux : Demux  Outputs=3
  Fourier : spsFourierLib/Fourier  Freq=60  n=1  InInit=[0, 0]  Ts=50e-6
  Gain : Gain  Gain=1/3
  Sum : Sum  Inputs=|+++
  Out1 : Outport  VectorParamsAs1DForOutWhenUnconnected=off
  wires:
  Sum/1 -> Gain/1
  Demux/3 -> Sum/3
  Demux/2 -> Sum/2
  Demux/1 -> Sum/1
  Fourier/1 -> Demux/1
  Gain/1 -> Out1/1
  In1/1 -> Fourier/1

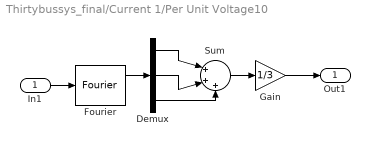
== system Thirtybussys_final/Current 1/Per Unit Voltage10 ==
  In1 : Inport
  Demux : Demux  Outputs=3
  Fourier : spsFourierLib/Fourier  Freq=60  n=1  InInit=[0, 0]  Ts=50e-6
  Gain : Gain  Gain=1/3
  Sum : Sum  Inputs=|+++
  Out1 : Outport  VectorParamsAs1DForOutWhenUnconnected=off
  wires:
  In1/1 -> Fourier/1
  Gain/1 -> Out1/1
  Fourier/1 -> Demux/1
  Demux/1 -> Sum/1
  Demux/2 -> Sum/2
  Demux/3 -> Sum/3
  Sum/1 -> Gain/1

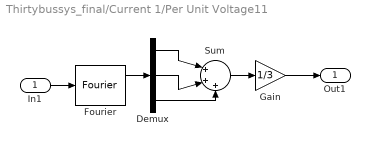
== system Thirtybussys_final/Current 1/Per Unit Voltage11 ==
  In1 : Inport
  Demux : Demux  Outputs=3
  Fourier : spsFourierLib/Fourier  Freq=60  n=1  InInit=[0, 0]  Ts=50e-6
  Gain : Gain  Gain=1/3
  Sum : Sum  Inputs=|+++
  Out1 : Outport  VectorParamsAs1DForOutWhenUnconnected=off
  wires:
  Sum/1 -> Gain/1
  Demux/3 -> Sum/3
  Demux/2 -> Sum/2
  Demux/1 -> Sum/1
  Fourier/1 -> Demux/1
  Gain/1 -> Out1/1
  In1/1 -> Fourier/1

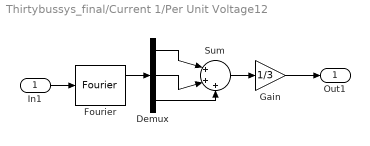
== system Thirtybussys_final/Current 1/Per Unit Voltage12 ==
  In1 : Inport
  Demux : Demux  Outputs=3
  Fourier : spsFourierLib/Fourier  Freq=60  n=1  InInit=[0, 0]  Ts=50e-6
  Gain : Gain  Gain=1/3
  Sum : Sum  Inputs=|+++
  Out1 : Outport  VectorParamsAs1DForOutWhenUnconnected=off
  wires:
  In1/1 -> Fourier/1
  Gain/1 -> Out1/1
  Fourier/1 -> Demux/1
  Demux/1 -> Sum/1
  Demux/2 -> Sum/2
  Demux/3 -> Sum/3
  Sum/1 -> Gain/1

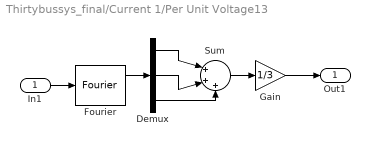
== system Thirtybussys_final/Current 1/Per Unit Voltage13 ==
  In1 : Inport
  Demux : Demux  Outputs=3
  Fourier : spsFourierLib/Fourier  Freq=60  n=1  InInit=[0, 0]  Ts=50e-6
  Gain : Gain  Gain=1/3
  Sum : Sum  Inputs=|+++
  Out1 : Outport  VectorParamsAs1DForOutWhenUnconnected=off
  wires:
  Sum/1 -> Gain/1
  Demux/3 -> Sum/3
  Demux/2 -> Sum/2
  Demux/1 -> Sum/1
  Fourier/1 -> Demux/1
  Gain/1 -> Out1/1
  In1/1 -> Fourier/1

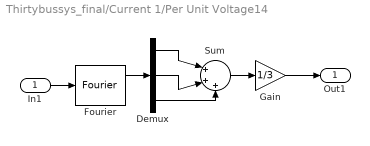
== system Thirtybussys_final/Current 1/Per Unit Voltage14 ==
  In1 : Inport
  Demux : Demux  Outputs=3
  Fourier : spsFourierLib/Fourier  Freq=60  n=1  InInit=[0, 0]  Ts=50e-6
  Gain : Gain  Gain=1/3
  Sum : Sum  Inputs=|+++
  Out1 : Outport  VectorParamsAs1DForOutWhenUnconnected=off
  wires:
  In1/1 -> Fourier/1
  Gain/1 -> Out1/1
  Fourier/1 -> Demux/1
  Demux/1 -> Sum/1
  Demux/2 -> Sum/2
  Demux/3 -> Sum/3
  Sum/1 -> Gain/1

== system Thirtybussys_final/Current 1/Per Unit Voltage15 ==
  In1 : Inport
  Demux : Demux  Outputs=3
  Fourier : spsFourierLib/Fourier  Freq=60  n=1  InInit=[0, 0]  Ts=50e-6
  Gain : Gain  Gain=1/3
  Sum : Sum  Inputs=|+++
  Out1 : Outport  VectorParamsAs1DForOutWhenUnconnected=off
  wires:
  Sum/1 -> Gain/1
  Demux/3 -> Sum/3
  Demux/2 -> Sum/2
  Demux/1 -> Sum/1
  Fourier/1 -> Demux/1
  Gain/1 -> Out1/1
  In1/1 -> Fourier/1

== system Thirtybussys_final/Current 1/Per Unit Voltage16 ==
  In1 : Inport
  Demux : Demux  Outputs=3
  Fourier : spsFourierLib/Fourier  Freq=60  n=1  InInit=[0, 0]  Ts=50e-6
  Gain : Gain  Gain=1/3
  Sum : Sum  Inputs=|+++
  Out1 : Outport  VectorParamsAs1DForOutWhenUnconnected=off
  wires:
  Sum/1 -> Gain/1
  Demux/3 -> Sum/3
  Demux/2 -> Sum/2
  Demux/1 -> Sum/1
  Fourier/1 -> Demux/1
  Gain/1 -> Out1/1
  In1/1 -> Fourier/1

== system Thirtybussys_final/Current 1/Per Unit Voltage17 ==
  In1 : Inport
  Demux : Demux  Outputs=3
  Fourier : spsFourierLib/Fourier  Freq=60  n=1  InInit=[0, 0]  Ts=50e-6
  Gain : Gain  Gain=1/3
  Sum : Sum  Inputs=|+++
  Out1 : Outport  VectorParamsAs1DForOutWhenUnconnected=off
  wires:
  In1/1 -> Fourier/1
  Gain/1 -> Out1/1
  Fourier/1 -> Demux/1
  Demux/1 -> Sum/1
  Demux/2 -> Sum/2
  Demux/3 -> Sum/3
  Sum/1 -> Gain/1

== system Thirtybussys_final/Current 1/Per Unit Voltage18 ==
  In1 : Inport
  Demux : Demux  Outputs=3
  Fourier : spsFourierLib/Fourier  Freq=60  n=1  InInit=[0, 0]  Ts=50e-6
  Gain : Gain  Gain=1/3
  Sum : Sum  Inputs=|+++
  Out1 : Outport  VectorParamsAs1DForOutWhenUnconnected=off
  wires:
  Sum/1 -> Gain/1
  Demux/3 -> Sum/3
  Demux/2 -> Sum/2
  Demux/1 -> Sum/1
  Fourier/1 -> Demux/1
  Gain/1 -> Out1/1
  In1/1 -> Fourier/1

== system Thirtybussys_final/Current 1/Per Unit Voltage19 ==
  In1 : Inport
  Demux : Demux  Outputs=3
  Fourier : spsFourierLib/Fourier  Freq=60  n=1  InInit=[0, 0]  Ts=50e-6
  Gain : Gain  Gain=1/3
  Sum : Sum  Inputs=|+++
  Out1 : Outport  VectorParamsAs1DForOutWhenUnconnected=off
  wires:
  In1/1 -> Fourier/1
  Gain/1 -> Out1/1
  Fourier/1 -> Demux/1
  Demux/1 -> Sum/1
  Demux/2 -> Sum/2
  Demux/3 -> Sum/3
  Sum/1 -> Gain/1

== system Thirtybussys_final/Current 1/Per Unit Voltage2 ==
  In1 : Inport
  Demux : Demux  Outputs=3
  Fourier : spsFourierLib/Fourier  Freq=60  n=1  InInit=[0, 0]  Ts=50e-6
  Gain : Gain  Gain=1/3
  Sum : Sum  Inputs=|+++
  Out1 : Outport  VectorParamsAs1DForOutWhenUnconnected=off
  wires:
  In1/1 -> Fourier/1
  Gain/1 -> Out1/1
  Fourier/1 -> Demux/1
  Demux/1 -> Sum/1
  Demux/2 -> Sum/2
  Demux/3 -> Sum/3
  Sum/1 -> Gain/1

== system Thirtybussys_final/Current 1/Per Unit Voltage20 ==
  In1 : Inport
  Demux : Demux  Outputs=3
  Fourier : spsFourierLib/Fourier  Freq=60  n=1  InInit=[0, 0]  Ts=50e-6
  Gain : Gain  Gain=1/3
  Sum : Sum  Inputs=|+++
  Out1 : Outport  VectorParamsAs1DForOutWhenUnconnected=off
  wires:
  Sum/1 -> Gain/1
  Demux/3 -> Sum/3
  Demux/2 -> Sum/2
  Demux/1 -> Sum/1
  Fourier/1 -> Demux/1
  Gain/1 -> Out1/1
  In1/1 -> Fourier/1

== system Thirtybussys_final/Current 1/Per Unit Voltage21 ==
  In1 : Inport
  Demux : Demux  Outputs=3
  Fourier : spsFourierLib/Fourier  Freq=60  n=1  InInit=[0, 0]  Ts=50e-6
  Gain : Gain  Gain=1/3
  Sum : Sum  Inputs=|+++
  Out1 : Outport  VectorParamsAs1DForOutWhenUnconnected=off
  wires:
  In1/1 -> Fourier/1
  Gain/1 -> Out1/1
  Fourier/1 -> Demux/1
  Demux/1 -> Sum/1
  Demux/2 -> Sum/2
  Demux/3 -> Sum/3
  Sum/1 -> Gain/1

== system Thirtybussys_final/Current 1/Per Unit Voltage22 ==
  In1 : Inport
  Demux : Demux  Outputs=3
  Fourier : spsFourierLib/Fourier  Freq=60  n=1  InInit=[0, 0]  Ts=50e-6
  Gain : Gain  Gain=1/3
  Sum : Sum  Inputs=|+++
  Out1 : Outport  VectorParamsAs1DForOutWhenUnconnected=off
  wires:
  Sum/1 -> Gain/1
  Demux/3 -> Sum/3
  Demux/2 -> Sum/2
  Demux/1 -> Sum/1
  Fourier/1 -> Demux/1
  Gain/1 -> Out1/1
  In1/1 -> Fourier/1

== system Thirtybussys_final/Current 1/Per Unit Voltage23 ==
  In1 : Inport
  Demux : Demux  Outputs=3
  Fourier : spsFourierLib/Fourier  Freq=60  n=1  InInit=[0, 0]  Ts=50e-6
  Gain : Gain  Gain=1/3
  Sum : Sum  Inputs=|+++
  Out1 : Outport  VectorParamsAs1DForOutWhenUnconnected=off
  wires:
  In1/1 -> Fourier/1
  Gain/1 -> Out1/1
  Fourier/1 -> Demux/1
  Demux/1 -> Sum/1
  Demux/2 -> Sum/2
  Demux/3 -> Sum/3
  Sum/1 -> Gain/1

== system Thirtybussys_final/Current 1/Per Unit Voltage24 ==
  In1 : Inport
  Demux : Demux  Outputs=3
  Fourier : spsFourierLib/Fourier  Freq=60  n=1  InInit=[0, 0]  Ts=50e-6
  Gain : Gain  Gain=1/3
  Sum : Sum  Inputs=|+++
  Out1 : Outport  VectorParamsAs1DForOutWhenUnconnected=off
  wires:
  In1/1 -> Fourier/1
  Gain/1 -> Out1/1
  Fourier/1 -> Demux/1
  Demux/1 -> Sum/1
  Demux/2 -> Sum/2
  Demux/3 -> Sum/3
  Sum/1 -> Gain/1

== system Thirtybussys_final/Current 1/Per Unit Voltage25 ==
  In1 : Inport
  Demux : Demux  Outputs=3
  Fourier : spsFourierLib/Fourier  Freq=60  n=1  InInit=[0, 0]  Ts=50e-6
  Gain : Gain  Gain=1/3
  Sum : Sum  Inputs=|+++
  Out1 : Outport  VectorParamsAs1DForOutWhenUnconnected=off
  wires:
  Sum/1 -> Gain/1
  Demux/3 -> Sum/3
  Demux/2 -> Sum/2
  Demux/1 -> Sum/1
  Fourier/1 -> Demux/1
  Gain/1 -> Out1/1
  In1/1 -> Fourier/1

== system Thirtybussys_final/Current 1/Per Unit Voltage26 ==
  In1 : Inport
  Demux : Demux  Outputs=3
  Fourier : spsFourierLib/Fourier  Freq=60  n=1  InInit=[0, 0]  Ts=50e-6
  Gain : Gain  Gain=1/3
  Sum : Sum  Inputs=|+++
  Out1 : Outport  VectorParamsAs1DForOutWhenUnconnected=off
  wires:
  In1/1 -> Fourier/1
  Gain/1 -> Out1/1
  Fourier/1 -> Demux/1
  Demux/1 -> Sum/1
  Demux/2 -> Sum/2
  Demux/3 -> Sum/3
  Sum/1 -> Gain/1

== system Thirtybussys_final/Current 1/Per Unit Voltage27 ==
  In1 : Inport
  Demux : Demux  Outputs=3
  Fourier : spsFourierLib/Fourier  Freq=60  n=1  InInit=[0, 0]  Ts=50e-6
  Gain : Gain  Gain=1/3
  Sum : Sum  Inputs=|+++
  Out1 : Outport  VectorParamsAs1DForOutWhenUnconnected=off
  wires:
  Sum/1 -> Gain/1
  Demux/3 -> Sum/3
  Demux/2 -> Sum/2
  Demux/1 -> Sum/1
  Fourier/1 -> Demux/1
  Gain/1 -> Out1/1
  In1/1 -> Fourier/1

== system Thirtybussys_final/Current 1/Per Unit Voltage28 ==
  In1 : Inport
  Demux : Demux  Outputs=3
  Fourier : spsFourierLib/Fourier  Freq=60  n=1  InInit=[0, 0]  Ts=50e-6
  Gain : Gain  Gain=1/3
  Sum : Sum  Inputs=|+++
  Out1 : Outport  VectorParamsAs1DForOutWhenUnconnected=off
  wires:
  In1/1 -> Fourier/1
  Gain/1 -> Out1/1
  Fourier/1 -> Demux/1
  Demux/1 -> Sum/1
  Demux/2 -> Sum/2
  Demux/3 -> Sum/3
  Sum/1 -> Gain/1

== system Thirtybussys_final/Current 1/Per Unit Voltage29 ==
  In1 : Inport
  Demux : Demux  Outputs=3
  Fourier : spsFourierLib/Fourier  Freq=60  n=1  InInit=[0, 0]  Ts=50e-6
  Gain : Gain  Gain=1/3
  Sum : Sum  Inputs=|+++
  Out1 : Outport  VectorParamsAs1DForOutWhenUnconnected=off
  wires:
  Sum/1 -> Gain/1
  Demux/3 -> Sum/3
  Demux/2 -> Sum/2
  Demux/1 -> Sum/1
  Fourier/1 -> Demux/1
  Gain/1 -> Out1/1
  In1/1 -> Fourier/1

== system Thirtybussys_final/Current 1/Per Unit Voltage3 ==
  In1 : Inport
  Demux : Demux  Outputs=3
  Fourier : spsFourierLib/Fourier  Freq=60  n=1  InInit=[0, 0]  Ts=50e-6
  Gain : Gain  Gain=1/3
  Sum : Sum  Inputs=|+++
  Out1 : Outport  VectorParamsAs1DForOutWhenUnconnected=off
  wires:
  Sum/1 -> Gain/1
  Demux/3 -> Sum/3
  Demux/2 -> Sum/2
  Demux/1 -> Sum/1
  Fourier/1 -> Demux/1
  Gain/1 -> Out1/1
  In1/1 -> Fourier/1

== system Thirtybussys_final/Current 1/Per Unit Voltage4 ==
  In1 : Inport
  Demux : Demux  Outputs=3
  Fourier : spsFourierLib/Fourier  Freq=60  n=1  InInit=[0, 0]  Ts=50e-6
  Gain : Gain  Gain=1/3
  Sum : Sum  Inputs=|+++
  Out1 : Outport  VectorParamsAs1DForOutWhenUnconnected=off
  wires:
  In1/1 -> Fourier/1
  Gain/1 -> Out1/1
  Fourier/1 -> Demux/1
  Demux/1 -> Sum/1
  Demux/2 -> Sum/2
  Demux/3 -> Sum/3
  Sum/1 -> Gain/1

== system Thirtybussys_final/Current 1/Per Unit Voltage5 ==
  In1 : Inport
  Demux : Demux  Outputs=3
  Fourier : spsFourierLib/Fourier  Freq=60  n=1  InInit=[0, 0]  Ts=50e-6
  Gain : Gain  Gain=1/3
  Sum : Sum  Inputs=|+++
  Out1 : Outport  VectorParamsAs1DForOutWhenUnconnected=off
  wires:
  Sum/1 -> Gain/1
  Demux/3 -> Sum/3
  Demux/2 -> Sum/2
  Demux/1 -> Sum/1
  Fourier/1 -> Demux/1
  Gain/1 -> Out1/1
  In1/1 -> Fourier/1

== system Thirtybussys_final/Current 1/Per Unit Voltage6 ==
  In1 : Inport
  Demux : Demux  Outputs=3
  Fourier : spsFourierLib/Fourier  Freq=60  n=1  InInit=[0, 0]  Ts=50e-6
  Gain : Gain  Gain=1/3
  Sum : Sum  Inputs=|+++
  Out1 : Outport  VectorParamsAs1DForOutWhenUnconnected=off
  wires:
  Sum/1 -> Gain/1
  Demux/3 -> Sum/3
  Demux/2 -> Sum/2
  Demux/1 -> Sum/1
  Fourier/1 -> Demux/1
  Gain/1 -> Out1/1
  In1/1 -> Fourier/1

== system Thirtybussys_final/Current 1/Per Unit Voltage7 ==
  In1 : Inport
  Demux : Demux  Outputs=3
  Fourier : spsFourierLib/Fourier  Freq=60  n=1  InInit=[0, 0]  Ts=50e-6
  Gain : Gain  Gain=1/3
  Sum : Sum  Inputs=|+++
  Out1 : Outport  VectorParamsAs1DForOutWhenUnconnected=off
  wires:
  In1/1 -> Fourier/1
  Gain/1 -> Out1/1
  Fourier/1 -> Demux/1
  Demux/1 -> Sum/1
  Demux/2 -> Sum/2
  Demux/3 -> Sum/3
  Sum/1 -> Gain/1

== system Thirtybussys_final/Current 1/Per Unit Voltage8 ==
  In1 : Inport
  Demux : Demux  Outputs=3
  Fourier : spsFourierLib/Fourier  Freq=60  n=1  InInit=[0, 0]  Ts=50e-6
  Gain : Gain  Gain=1/3
  Sum : Sum  Inputs=|+++
  Out1 : Outport  VectorParamsAs1DForOutWhenUnconnected=off
  wires:
  Sum/1 -> Gain/1
  Demux/3 -> Sum/3
  Demux/2 -> Sum/2
  Demux/1 -> Sum/1
  Fourier/1 -> Demux/1
  Gain/1 -> Out1/1
  In1/1 -> Fourier/1

== system Thirtybussys_final/Current 1/Per Unit Voltage9 ==
  In1 : Inport
  Demux : Demux  Outputs=3
  Fourier : spsFourierLib/Fourier  Freq=60  n=1  InInit=[0, 0]  Ts=50e-6
  Gain : Gain  Gain=1/3
  Sum : Sum  Inputs=|+++
  Out1 : Outport  VectorParamsAs1DForOutWhenUnconnected=off
  wires:
  In1/1 -> Fourier/1
  Gain/1 -> Out1/1
  Fourier/1 -> Demux/1
  Demux/1 -> Sum/1
  Demux/2 -> Sum/2
  Demux/3 -> Sum/3
  Sum/1 -> Gain/1

== system Thirtybussys_final/Voltage /Per Unit Voltage ==
  In1 : Inport
  Demux : Demux  Outputs=3
  Fourier : spsFourierLib/Fourier  Freq=60  n=1  InInit=[0, 0]  Ts=50e-6
  Gain : Gain  Gain=1/3
  Sum : Sum  Inputs=|+++
  Out1 : Outport  VectorParamsAs1DForOutWhenUnconnected=off
  wires:
  In1/1 -> Fourier/1
  Gain/1 -> Out1/1
  Fourier/1 -> Demux/1
  Demux/1 -> Sum/1
  Demux/2 -> Sum/2
  Demux/3 -> Sum/3
  Sum/1 -> Gain/1

== system Thirtybussys_final/Voltage /Per Unit Voltage1 ==
  In1 : Inport
  Demux : Demux  Outputs=3
  Fourier : spsFourierLib/Fourier  Freq=60  n=1  InInit=[0, 0]  Ts=50e-6
  Gain : Gain  Gain=1/3
  Sum : Sum  Inputs=|+++
  Out1 : Outport  VectorParamsAs1DForOutWhenUnconnected=off
  wires:
  Sum/1 -> Gain/1
  Demux/3 -> Sum/3
  Demux/2 -> Sum/2
  Demux/1 -> Sum/1
  Fourier/1 -> Demux/1
  Gain/1 -> Out1/1
  In1/1 -> Fourier/1

== system Thirtybussys_final/Voltage /Per Unit Voltage10 ==
  In1 : Inport
  Demux : Demux  Outputs=3
  Fourier : spsFourierLib/Fourier  Freq=60  n=1  InInit=[0, 0]  Ts=50e-6
  Gain : Gain  Gain=1/3
  Sum : Sum  Inputs=|+++
  Out1 : Outport  VectorParamsAs1DForOutWhenUnconnected=off
  wires:
  In1/1 -> Fourier/1
  Gain/1 -> Out1/1
  Fourier/1 -> Demux/1
  Demux/1 -> Sum/1
  Demux/2 -> Sum/2
  Demux/3 -> Sum/3
  Sum/1 -> Gain/1

== system Thirtybussys_final/Voltage /Per Unit Voltage11 ==
  In1 : Inport
  Demux : Demux  Outputs=3
  Fourier : spsFourierLib/Fourier  Freq=60  n=1  InInit=[0, 0]  Ts=50e-6
  Gain : Gain  Gain=1/3
  Sum : Sum  Inputs=|+++
  Out1 : Outport  VectorParamsAs1DForOutWhenUnconnected=off
  wires:
  Sum/1 -> Gain/1
  Demux/3 -> Sum/3
  Demux/2 -> Sum/2
  Demux/1 -> Sum/1
  Fourier/1 -> Demux/1
  Gain/1 -> Out1/1
  In1/1 -> Fourier/1

== system Thirtybussys_final/Voltage /Per Unit Voltage12 ==
  In1 : Inport
  Demux : Demux  Outputs=3
  Fourier : spsFourierLib/Fourier  Freq=60  n=1  InInit=[0, 0]  Ts=50e-6
  Gain : Gain  Gain=1/3
  Sum : Sum  Inputs=|+++
  Out1 : Outport  VectorParamsAs1DForOutWhenUnconnected=off
  wires:
  In1/1 -> Fourier/1
  Gain/1 -> Out1/1
  Fourier/1 -> Demux/1
  Demux/1 -> Sum/1
  Demux/2 -> Sum/2
  Demux/3 -> Sum/3
  Sum/1 -> Gain/1

== system Thirtybussys_final/Voltage /Per Unit Voltage13 ==
  In1 : Inport
  Demux : Demux  Outputs=3
  Fourier : spsFourierLib/Fourier  Freq=60  n=1  InInit=[0, 0]  Ts=50e-6
  Gain : Gain  Gain=1/3
  Sum : Sum  Inputs=|+++
  Out1 : Outport  VectorParamsAs1DForOutWhenUnconnected=off
  wires:
  Sum/1 -> Gain/1
  Demux/3 -> Sum/3
  Demux/2 -> Sum/2
  Demux/1 -> Sum/1
  Fourier/1 -> Demux/1
  Gain/1 -> Out1/1
  In1/1 -> Fourier/1

== system Thirtybussys_final/Voltage /Per Unit Voltage14 ==
  In1 : Inport
  Demux : Demux  Outputs=3
  Fourier : spsFourierLib/Fourier  Freq=60  n=1  InInit=[0, 0]  Ts=50e-6
  Gain : Gain  Gain=1/3
  Sum : Sum  Inputs=|+++
  Out1 : Outport  VectorParamsAs1DForOutWhenUnconnected=off
  wires:
  In1/1 -> Fourier/1
  Gain/1 -> Out1/1
  Fourier/1 -> Demux/1
  Demux/1 -> Sum/1
  Demux/2 -> Sum/2
  Demux/3 -> Sum/3
  Sum/1 -> Gain/1

== system Thirtybussys_final/Voltage /Per Unit Voltage15 ==
  In1 : Inport
  Demux : Demux  Outputs=3
  Fourier : spsFourierLib/Fourier  Freq=60  n=1  InInit=[0, 0]  Ts=50e-6
  Gain : Gain  Gain=1/3
  Sum : Sum  Inputs=|+++
  Out1 : Outport  VectorParamsAs1DForOutWhenUnconnected=off
  wires:
  Sum/1 -> Gain/1
  Demux/3 -> Sum/3
  Demux/2 -> Sum/2
  Demux/1 -> Sum/1
  Fourier/1 -> Demux/1
  Gain/1 -> Out1/1
  In1/1 -> Fourier/1

== system Thirtybussys_final/Voltage /Per Unit Voltage16 ==
  In1 : Inport
  Demux : Demux  Outputs=3
  Fourier : spsFourierLib/Fourier  Freq=60  n=1  InInit=[0, 0]  Ts=50e-6
  Gain : Gain  Gain=1/3
  Sum : Sum  Inputs=|+++
  Out1 : Outport  VectorParamsAs1DForOutWhenUnconnected=off
  wires:
  Sum/1 -> Gain/1
  Demux/3 -> Sum/3
  Demux/2 -> Sum/2
  Demux/1 -> Sum/1
  Fourier/1 -> Demux/1
  Gain/1 -> Out1/1
  In1/1 -> Fourier/1

== system Thirtybussys_final/Voltage /Per Unit Voltage17 ==
  In1 : Inport
  Demux : Demux  Outputs=3
  Fourier : spsFourierLib/Fourier  Freq=60  n=1  InInit=[0, 0]  Ts=50e-6
  Gain : Gain  Gain=1/3
  Sum : Sum  Inputs=|+++
  Out1 : Outport  VectorParamsAs1DForOutWhenUnconnected=off
  wires:
  In1/1 -> Fourier/1
  Gain/1 -> Out1/1
  Fourier/1 -> Demux/1
  Demux/1 -> Sum/1
  Demux/2 -> Sum/2
  Demux/3 -> Sum/3
  Sum/1 -> Gain/1

== system Thirtybussys_final/Voltage /Per Unit Voltage18 ==
  In1 : Inport
  Demux : Demux  Outputs=3
  Fourier : spsFourierLib/Fourier  Freq=60  n=1  InInit=[0, 0]  Ts=50e-6
  Gain : Gain  Gain=1/3
  Sum : Sum  Inputs=|+++
  Out1 : Outport  VectorParamsAs1DForOutWhenUnconnected=off
  wires:
  Sum/1 -> Gain/1
  Demux/3 -> Sum/3
  Demux/2 -> Sum/2
  Demux/1 -> Sum/1
  Fourier/1 -> Demux/1
  Gain/1 -> Out1/1
  In1/1 -> Fourier/1
